simulink model "generator_simulation"  (R2019a)
settings: Solver=FixedStepAuto  StartTime=0.0  StopTime=600  FixedStep=Ts  MaxStep=Ts  RelTol=1e-3
PreLoadFcn:
  | Ts = Ts;
values from neighbouring files (symbols this model uses):
  alpha = 0    [parameters.m]
  Area = 1.13    [parameters.m]
  c_d = 0.5    [parameters.m]
  f = 0.018    [parameters.m]
  g = 9.81    [parameters.m]
  I_initial = v_desired/(R_bx)    (= 0)    [parameters.m]
  Jb = (m_b)*((R_bxb)^2)    (= 41.86125)    [parameters.m]
  Jx = (m_x)*((R_bx)^2)    (= 29.64574716)    [parameters.m]
  m_b = 450    [parameters.m]
  p = 1.204    [parameters.m]
  R_bx = 0.4318    [parameters.m]
  R_bxb = 0.305    [parameters.m]
libraries: powerlib x13, simulink x6
settings Model: EnablePacing=on  Creator=Phuc  LastModifiedBy=Dinh Ngoc Quy
settings SolverCC: AlgebraicLoopSolver=LineSearch
settings DataIOCC: ReturnWorkspaceOutputs=off
settings DebuggingCC: AlgebraicLoopMsg=none  ArithmeticOperatorsInVariantConditions=warning
settings SFSimCC: SimUseLocalCustomCode=off
settings RTWCC: RTWUseLocalCustomCode=off

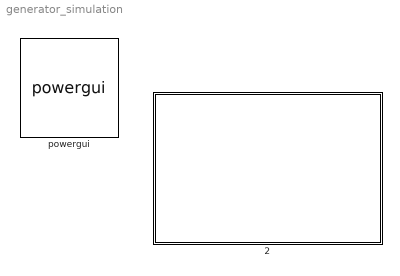
== system generator_simulation ==
  2 : Subsystem
      mask Display:
      | image('motorelec.jpg')
      | port_label('input',1,'w (rad/s)')
  powergui : powerlib/powergui  SimulationMode=Discrete  SampleTime=Ts  frequency=60  Iterations=50  frequencyindice=50  Pbase=100e6  ErrMax=1e-4  UnitsV=kV  UnitsW=MW  buscounter=0  FunctionMessages=off  echomessages=off  EnableUseOfTLC=off  CurrentSourceSwitches=off  DisableSnubberDevices=off  DisableRonSwitches=off  DisableVfSwitches=off  DisplayEquations=off  AutomaticDiscreteSolvers=off  SolverType=Tustin/Backward Euler (TBE)  Interpol=off  ExternalGateDelay=off  methode=off  Ts=100  x0status=blocks  SPID=off  SwTol=0  HookPort=off  NonlinearTolerance=0  nMaxIteration=15  ContinueOnMaxIteration=off  RestoreLinks=warning  ResistiveCurrentMeasurement=off  Frange=[0:2:500]  Ylog=off  Xlog=on  ShowGrid=off  save=off  variable=ZData  structure=0  ZoomFFT=on  StartTime=0.0  cycles=1  DisplayStyle=1  fundamental=60  FreqAxis=off  MaxFrequency=1000  frequencyindicesteady=1  RmsSteady=1  display=off
      settings: SourceProductName=Simscape Electrical

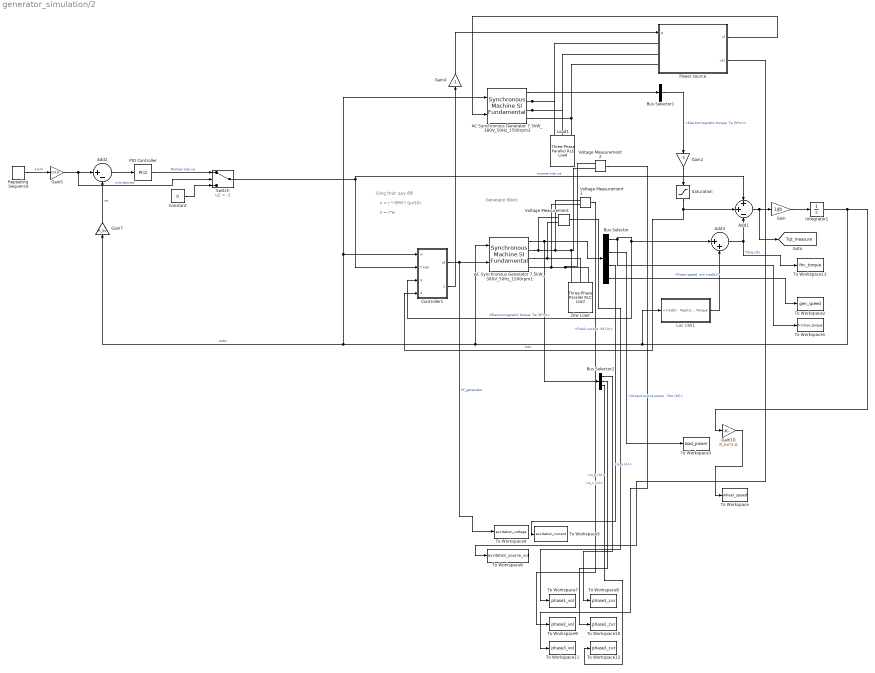
== system generator_simulation/2 ==
  note: Generator Block
  note: Công thức quy đổi
  note: v = r * RPM * (pi/30)
  note: v = r*w
  2kw Load : powerlib/Elements/Three-Phase Parallel RLC Load  LConnTagsString=A|B|C  Configuration=Y (grounded)  NominalVoltage=72  Vabc=[1e3 1e3 1e3]  Vabcp=[1e3 1e3 1e3]  NominalFrequency=50  UnbalancedPower=off  ActivePower=1000  InductivePower=0  CapacitivePower=0  Pabc=[10e3 9e3 11e3]  QLabc=[100 90 110]  QCabc=[100 90 110]  Pabcp=[10e3 9e3 11e3]  QLabcp=[100 90 110]  QCabcp=[100 90 110]  Measurements=None  LoadType=constant Z
      settings: SourceProductName=Simscape Electrical
  AC Synchronous Generator 7.5kW_380V_50Hz_1500rpm1 : powerlib/Machines/Synchronous Machine SI Fundamental  PresetModel=No  MechanicalLoad=Speed w  ShowDetailedParameters=on  RotorType=Salient-pole  Units=SI fundamental parameters  MeasurementBus=off  NominalParameters=[7500 220 50 2]  Stator=[1.62 0.004527 0.1086 0.05175]  Field=[1.208 0.01132]  Dampers2=[ 0.0664, 1.387e-3, 0.0292, 6.896e-4, 7.907e-3, 2.477e-3]  Dampers1=[3.142 0.007334 4.772 0.01015]  Mechanical=[0.0923 0.009 2]  PolePairs=2  InitialConditions="[ 0  0  0  0  0  0  0  0 0]"  SetSaturation=off  Saturation=[695.64,774.7,917.5,1001.6,1082.2,1175.9,1293.6,1430.2,1583.7;9660,10623,12243,13063,13757,14437,15180,15890,16567]  DisplayVfd=off  LoadFlowParameters=[1,0,0,0,0]  TsPowergui=0  TsBlock=-1  IterativeModel=Trapezoidal non iterative  IterativeDiscreteModel=Trapezoidal non iterative  BusType=swing  Pref=0  Qref=0  Qmin=-inf  Qmax=inf  PLF=0  QLF=0
      settings: SourceProductName=Simscape Electrical  SourceProductBaseCode=PS
  AC Synchronous Generator 7.5kW_380V_50Hz_1500rpm2 : powerlib/Machines/Synchronous Machine SI Fundamental  PresetModel=No  MechanicalLoad=Speed w  ShowDetailedParameters=on  RotorType=Salient-pole  Units=SI fundamental parameters  MeasurementBus=off  NominalParameters=[7500 220 50 2]  Stator=[1.62 0.004527 0.1086 0.05175]  Field=[1.208 0.01132]  Dampers2=[ 0.0664, 1.387e-3, 0.0292, 6.896e-4, 7.907e-3, 2.477e-3]  Dampers1=[3.142 0.007334 4.772 0.01015]  Mechanical=[0.0923 0.009 2]  PolePairs=2  InitialConditions="[ 0  0  0  0  0  0  0  0 0]"  SetSaturation=off  Saturation=[695.64,774.7,917.5,1001.6,1082.2,1175.9,1293.6,1430.2,1583.7;9660,10623,12243,13063,13757,14437,15180,15890,16567]  DisplayVfd=off  LoadFlowParameters=[1,0,0,0,0]  TsPowergui=0  TsBlock=-1  IterativeModel=Trapezoidal non iterative  IterativeDiscreteModel=Trapezoidal non iterative  BusType=swing  Pref=0  Qref=0  Qmin=-inf  Qmax=inf  PLF=0  QLF=0
      settings: SourceProductName=Simscape Electrical  SourceProductBaseCode=PS
  Add1 : Sum  Inputs=++-
  Add2 : Sum  Inputs=|+-
  Add3 : Sum  Inputs=|++
  Bus Selector : BusSelector  OutputSignals="Mechanical.Electromagnetic torque  Te (N*m),Output active power   Peo (W),dq0 components.Field current  ifd (A),Mechanical.Rotor speed  wm (rad/s)"
  Bus Selector1 : BusSelector  OutputSignals="Mechanical.Electromagnetic torque  Te (N*m)"
  Bus Selector2 : BusSelector  OutputSignals=Stator current.is_a (A),Stator current.is_b (A),Stator current.is_c (A)
  Constant : Constant  Value=0
  Controller1 : Subsystem
  Gain : Gain  Gain=1/Jb
  Gain10 : Gain  Gain=R_bx*3.6
  Gain2 : Gain  Gain=-1
  Gain4 : Gain  Gain=-1
  Gain5 : Gain  Gain=1/3.6
  Gain7 : Gain  Gain=R_bx
  Integrator1 : Integrator  InitialCondition=I_initial  LimitOutput=on  LowerSaturationLimit=0  ContinuousStateAttributes='velocity'
  Load1 : powerlib/Elements/Three-Phase Parallel RLC Load  LConnTagsString=A|B|C  Configuration=Y (grounded)  NominalVoltage=72  Vabc=[1e3 1e3 1e3]  Vabcp=[1e3 1e3 1e3]  NominalFrequency=50  UnbalancedPower=off  ActivePower=50  InductivePower=0  CapacitivePower=0  Pabc=[10e3 9e3 11e3]  QLabc=[100 90 110]  QCabc=[100 90 110]  Pabcp=[10e3 9e3 11e3]  QLabcp=[100 90 110]  QCabcp=[100 90 110]  Measurements=None  LoadType=constant Z
      settings: SourceProductName=Simscape Electrical
  Luc can1 : Subsystem
  PID Controller : simulink/Continuous/PID Controller  Controller=PI  Form=Ideal  TimeDomain=Discrete-time  SampleTime=-1  IntegratorMethod=Forward Euler  FilterMethod=Forward Euler  ControllerParametersSource=internal  P=435.0333770128  I=0.175017866772017  D=0  UseFilter=on  N=100  TunerSelectOption=Transfer Function Based (PID Tuner App)  InitialConditionSource=internal  InitialConditionForIntegrator=0  InitialConditionForFilter=0  DifferentiatorICPrevScaledInput=0  ExternalReset=none  TrackingMode=off  Kt=1  LimitOutput=off  UpperSaturationLimit=inf  LowerSaturationLimit=-inf  LinearizeAsGain=on  AntiWindupMode=none  Kb=1  POutMin=[]  POutMax=[]  IOutMin=[]  IOutMax=[]  DOutMin=[]  DOutMax=[]  NOutMin=[]  NOutMax=[]  SumOutMin=[]  SumOutMax=[]  SaturationOutMin=[]  SaturationOutMax=[]  PParamMin=[]  PParamMax=[]  IParamMin=[]  IParamMax=[]  DParamMin=[]  DParamMax=[]  NParamMin=[]  NParamMax=[]  KbParamMin=[]  KbParamMax=[]  KtParamMin=[]  KtParamMax=[]  KbOutMin=[]  KbOutMax=[]  KtOutMin=[]  KtOutMax=[]  IntegratorOutMin=[]  IntegratorOutMax=[]  FilterOutMin=[]  FilterOutMax=[]  SumI1OutMin=[]  SumI1OutMax=[]  SumI2OutMin=[]  SumI2OutMax=[]  SumI3OutMin=[]  SumI3OutMax=[]  SumI4OutMin=[]  SumI4OutMax=[]  SumDOutMin=[]  SumDOutMax=[]  DifferentiatorOutMin=[]  DifferentiatorOutMax=[]  FilterDiffOutCoefMin=[]  FilterDiffOutCoefMax=[]  ReciprocalOutMin=[]  ReciprocalOutMax=[]  SumDenOutMin=[]  SumDenOutMax=[]  SumNumOutMin=[]  SumNumOutMax=[]  DivideOutMin=[]  DivideOutMax=[]  IntegratorContinuousStateAttributes=''  IntegratorStateMustResolveToSignalObject=off  IntegratorRTWStateStorageClass=Auto  FilterContinuousStateAttributes=''  FilterStateMustResolveToSignalObject=off  FilterRTWStateStorageClass=Auto  ParallelPVariant=Passthrough  IdealPVariant=InternalParameters  IVariant=InternalParameters  DVariant=Disabled  IntegratorVariant=Discrete  SatVariant=Disabled  AWVariant=Passthrough  PCopyVariant=Disabled  TRVariant=Disabled  FdbkBlocksVariant=Forward  IdealPFdbkVariant=Disabled  SatFdbkVariant=Disabled  DerivativeFilterVariant=Disabled  NVariant=Disabled  NCopyVariant=Disabled_SignalSpec  FilterICVariant=Disabled  IntegratorICVariant=InternalICs  ExternalResetVariant=Disabled  TRSumVariant=Passthrough  SumFdbkVariant=Disabled  SumVariant=Sum_PI
  Power source : Subsystem
  Repeating Sequence : simulink/Sources/Repeating Sequence  rep_seq_t=DriveCycle_time  rep_seq_y=DriveCycle_speed
  Saturation : Saturate  UpperLimit=inf  LowerLimit=0
  Switch : Switch  Criteria=u2 > Threshold  Threshold=-1
  To Workspace : ToWorkspace  VariableName=wheel_speed  SaveFormat=Timeseries  SampleTime=1
  To Workspace1 : ToWorkspace  VariableName=friction_torque  SaveFormat=Timeseries  SampleTime=1
  To Workspace10 : ToWorkspace  VariableName=phase2_cur  SaveFormat=Timeseries  SampleTime=1
  To Workspace11 : ToWorkspace  VariableName=phase3_vol  SaveFormat=Timeseries  SampleTime=1
  To Workspace12 : ToWorkspace  VariableName=phase3_cur  SaveFormat=Timeseries  SampleTime=1
  To Workspace13 : ToWorkspace  VariableName=fric_torque  SaveFormat=Timeseries  SampleTime=1
  To Workspace2 : ToWorkspace  VariableName=gen_speed  SaveFormat=Timeseries  SampleTime=1
  To Workspace3 : ToWorkspace  VariableName=load_power  SaveFormat=Timeseries  SampleTime=1
  To Workspace4 : ToWorkspace  VariableName=excitation_voltage  SaveFormat=Timeseries  SampleTime=1
  To Workspace5 : ToWorkspace  VariableName=excitation_current  SaveFormat=Timeseries  SampleTime=1
  To Workspace6 : ToWorkspace  VariableName=excitation_source_vol  SaveFormat=Timeseries  SampleTime=1
  To Workspace7 : ToWorkspace  VariableName=phase1_vol  SaveFormat=Timeseries  SampleTime=1
  To Workspace8 : ToWorkspace  VariableName=phase1_cur  SaveFormat=Timeseries  SampleTime=1
  To Workspace9 : ToWorkspace  VariableName=phase2_vol  SaveFormat=Timeseries  SampleTime=1
  Voltage Measurement : powerlib/Measurements/Voltage Measurement  PhasorSimulation=off  OutputType=Complex  PSBequivalent=0
      settings: SourceProductName=Simscape Electrical
  Voltage Measurement1 : powerlib/Measurements/Voltage Measurement  PhasorSimulation=off  OutputType=Complex  PSBequivalent=0
      settings: SourceProductName=Simscape Electrical
  Voltage Measurement2 : powerlib/Measurements/Voltage Measurement  PhasorSimulation=off  OutputType=Complex  PSBequivalent=0
      settings: SourceProductName=Simscape Electrical
  tag scope: Tqt_measure=global
  wires:
  Saturation/1 -> Add1/2, Controller1/4(T_motor)  "kéo"
  Integrator1/1 -> Gain10/1, Luc can1/1(v (rad/s)), AC Synchronous Generator 7.5kW_380V_50Hz_1500rpm1/1, Gain7/1, AC Synchronous Generator 7.5kW_380V_50Hz_1500rpm2/1, Controller1/1(w)  "rad/s"
  Gain2/1 -> Saturation/1
  Bus Selector1/1 -> Gain2/1  "<Electromagnetic torque  Te (N*m)>"
  AC Synchronous Generator 7.5kW_380V_50Hz_1500rpm2/1 -> Bus Selector1/1
  Add3/1 -> Add1/3, To Workspace13/1  "Tổng cản"
  Luc can1/1(Resitive Torque) -> Add3/2
  Add1/1 -> [Tqt_measure], Gain/1
  Bus Selector/1 -> Controller1/3(T_measured), Add3/1, To Workspace1/1  "<Electromagnetic torque  Te (N*m)>"
  Gain/1 -> Integrator1/1
  AC Synchronous Generator 7.5kW_380V_50Hz_1500rpm1/1 -> Bus Selector2/1, Bus Selector/1
  Controller1/1(Vf) -> To Workspace4/1, AC Synchronous Generator 7.5kW_380V_50Hz_1500rpm1/2  "Vf_generator"
  Power source/1(vf) -> AC Synchronous Generator 7.5kW_380V_50Hz_1500rpm2/2
  Repeating Sequence/1 -> Gain5/1  "km/h"
  Add2/1 -> PID Controller/1
  Gain7/1 -> Add2/2  "xe"
  Gain5/1 -> Switch/2, Add2/1  "m/s desired"
  Switch/1 -> Add1/1, Controller1/2(T kéo)  "momen kéo xe"
  Constant/1 -> Switch/3
  PID Controller/1 -> Switch/1  "Momen kéo xe"
  Controller1/2(Vf_motor) -> Gain4/1
  Gain4/1 -> Power source/1(g)
  Bus Selector/2 -> To Workspace3/1  "<Output active power   Peo (W)>"
  Gain10/1 -> To Workspace/1
  Bus Selector/3 -> To Workspace5/1  "<Field current  ifd (A)>"
  Power source/2(vf1) -> To Workspace6/1
  Bus Selector2/1 -> To Workspace8/1  "<is_a (A)>"
  Bus Selector2/2 -> To Workspace10/1  "<is_b (A)>"
  Bus Selector2/3 -> To Workspace12/1  "<is_c (A)>"
  Voltage Measurement/1 -> To Workspace7/1
  Voltage Measurement1/1 -> To Workspace9/1
  Voltage Measurement2/1 -> To Workspace11/1
  Bus Selector/4 -> To Workspace2/1  "<Rotor speed  wm (rad/s)>"
  connections:
  AC Synchronous Generator 7.5kW_380V_50Hz_1500rpm2/RConn3 -- Power source/LConn3 -- Load1/LConn3
  AC Synchronous Generator 7.5kW_380V_50Hz_1500rpm2/RConn2 -- Power source/LConn2 -- Load1/LConn2
  AC Synchronous Generator 7.5kW_380V_50Hz_1500rpm2/RConn1 -- Power source/LConn1 -- Load1/LConn1
  AC Synchronous Generator 7.5kW_380V_50Hz_1500rpm1/RConn2 -- Voltage Measurement/LConn2 -- 2kw Load/LConn2
  2kw Load/LConn3 -- Voltage Measurement2/LConn1 -- Voltage Measurement1/LConn2 -- AC Synchronous Generator 7.5kW_380V_50Hz_1500rpm1/RConn3
  AC Synchronous Generator 7.5kW_380V_50Hz_1500rpm1/RConn1 -- Voltage Measurement/LConn1 -- Voltage Measurement1/LConn1 -- Voltage Measurement2/LConn2 -- 2kw Load/LConn1

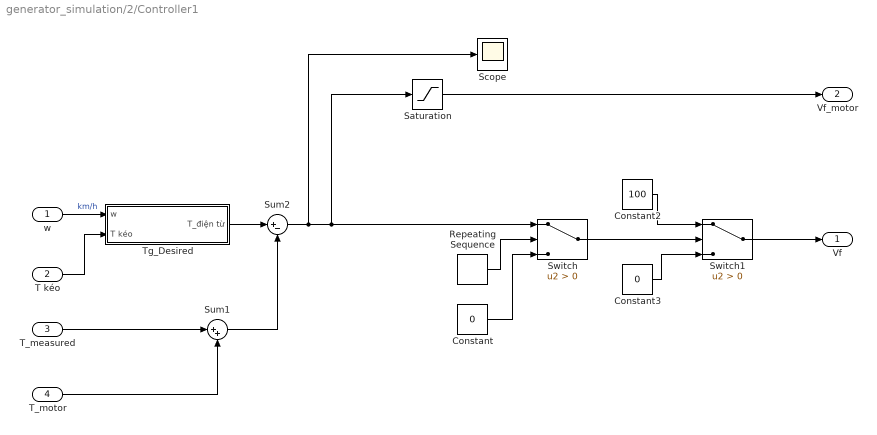
== system generator_simulation/2/Controller1 ==
  w : Inport
  T kéo : Inport  Port=2
  T_measured : Inport  Port=3
  T_motor : Inport  Port=4
  Constant : Constant  Value=0
  Constant2 : Constant  Value=100
  Constant3 : Constant  Value=0
  Repeating Sequence : simulink/Sources/Repeating Sequence  rep_seq_t=DriveCycle_time  rep_seq_y=DriveCycle_speed
  Saturation : Saturate  UpperLimit=0  LowerLimit=-inf
  Scope : Scope
  Sum1 : Sum  Inputs=|++
  Sum2 : Sum  Inputs=|+-
  Switch : Switch  Criteria=u2 > Threshold
  Switch1 : Switch  Criteria=u2 > Threshold
  Tg_Desired : Subsystem
  Vf : Outport
  Vf_motor : Outport  Port=2
  wires:
  Sum1/1 -> Sum2/2
  T_motor/1 -> Sum1/2
  T_measured/1 -> Sum1/1
  Sum2/1 -> Scope/1, Saturation/1, Switch/1
  Tg_Desired/1(T_điện từ) -> Sum2/1
  Switch1/1 -> Vf/1
  Constant3/1 -> Switch1/3
  Constant2/1 -> Switch1/1
  T kéo/1 -> Tg_Desired/2(T kéo)
  w/1 -> Tg_Desired/1(w)  "km/h"
  Constant/1 -> Switch/3
  Switch/1 -> Switch1/2
  Repeating Sequence/1 -> Switch/2
  Saturation/1 -> Vf_motor/1

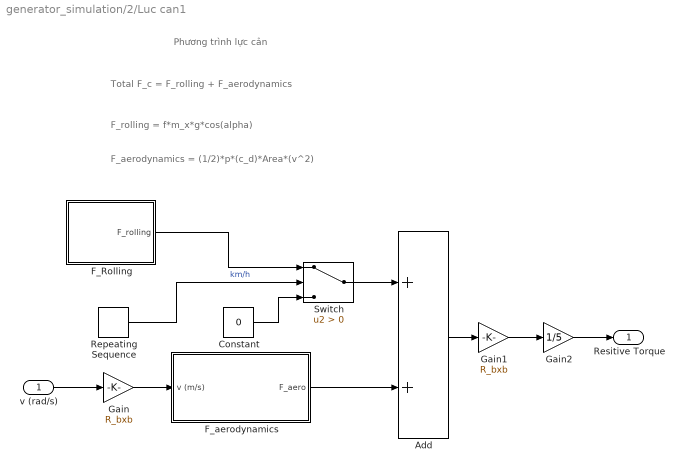
== system generator_simulation/2/Luc can1 ==
  note: Phương trình lực cản
  note: F_aerodynamics = (1/2)*p*(c_d)*Area*(v^2)
  note: F_rolling = f*m_x*g*cos(alpha)
  note: Total F_c = F_rolling + F_aerodynamics
  v (rad/s) : Inport
  Add : Sum
  Constant : Constant  Value=0
  F_Rolling : Subsystem
  F_aerodynamics : Subsystem
  Gain : Gain  Gain=R_bxb
  Gain1 : Gain  Gain=R_bxb
  Gain2 : Gain  Gain=1/5
  Repeating Sequence : simulink/Sources/Repeating Sequence  rep_seq_t=DriveCycle_time  rep_seq_y=DriveCycle_speed
  Switch : Switch  Criteria=u2 > Threshold
  Resitive Torque : Outport
  wires:
  Gain1/1 -> Gain2/1
  Gain/1 -> F_aerodynamics/1(v (m/s))
  Add/1 -> Gain1/1
  v (rad/s)/1 -> Gain/1
  Gain2/1 -> Resitive Torque/1
  F_aerodynamics/1(F_aero) -> Add/2
  Repeating Sequence/1 -> Switch/2  "km/h"
  Constant/1 -> Switch/3
  F_Rolling/1(F_rolling) -> Switch/1
  Switch/1 -> Add/1

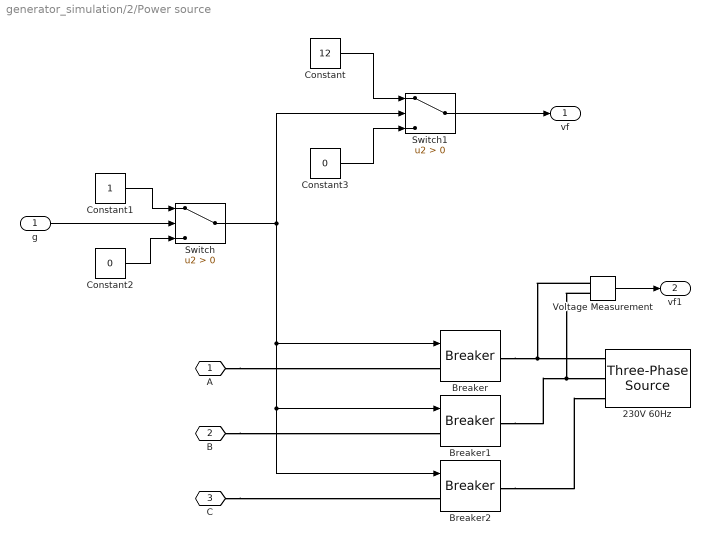
== system generator_simulation/2/Power source ==
  g : Inport
  230V 60Hz : powerlib/Electrical Sources/Three-Phase Source  InternalConnection=Yg  VoltagePhases=off  Voltage=72  PhaseAngle=0  Voltage_phases=[25e3 25e3 25e3]/sqrt(3)  PhaseAngles_phases=[0 -120 +120]  Frequency=50  NonIdealSource=on  SpecifyImpedance=off  Resistance=0.0002  Inductance=0.05e-3  ShortCircuitLevel=100e6  BaseVoltage=72  XRratio=7  BusType=swing  Pref=0  Qref=0  Prefabc=[10e3, 10e3, 10e3]  Qrefabc=[0, 0, 0]  Qmin=-inf  Qmax=inf
      settings: SourceProductName=Simscape Electrical
  Breaker : powerlib/Elements/Breaker  InitialState=0  SwitchingTimes="[1/60  5/60]"  External=on  BreakerResistance=0.01  SnubberResistance=1e6  SnubberCapacitance=inf  Measurements=None  MoreParameters=on  NoBreakLoop=off
      settings: SourceProductName=Simscape Electrical
  Breaker1 : powerlib/Elements/Breaker  InitialState=0  SwitchingTimes="[1/60  5/60]"  External=on  BreakerResistance=0.01  SnubberResistance=1e6  SnubberCapacitance=inf  Measurements=None  MoreParameters=on  NoBreakLoop=off
      settings: SourceProductName=Simscape Electrical
  Breaker2 : powerlib/Elements/Breaker  InitialState=0  SwitchingTimes="[1/60  5/60]"  External=on  BreakerResistance=0.01  SnubberResistance=1e6  SnubberCapacitance=inf  Measurements=None  MoreParameters=on  NoBreakLoop=off
      settings: SourceProductName=Simscape Electrical
  Constant : Constant  Value=12
  Constant1 : Constant
  Constant2 : Constant  Value=0
  Constant3 : Constant  Value=0
  Switch : Switch  Criteria=u2 > Threshold
  Switch1 : Switch  Criteria=u2 > Threshold
  Voltage Measurement : powerlib/Measurements/Voltage Measurement  PhasorSimulation=off  OutputType=Complex  PSBequivalent=0
      settings: SourceProductName=Simscape Electrical
  A : PMIOPort  Side=Left
  B : PMIOPort  Port=2  Side=Left
  C : PMIOPort  Port=3  Side=Left
  vf : Outport
  vf1 : Outport  Port=2
  wires:
  Switch1/1 -> vf/1
  Constant3/1 -> Switch1/3
  Constant/1 -> Switch1/1
  g/1 -> Switch/2
  Constant2/1 -> Switch/3
  Constant1/1 -> Switch/1
  Switch/1 -> Switch1/2, Breaker/1, Breaker1/1, Breaker2/1
  Voltage Measurement/1 -> vf1/1
  connections:
  B/RConn1 -- Breaker1/LConn1
  C/RConn1 -- Breaker2/LConn1
  A/RConn1 -- Breaker/LConn1
  Breaker1/RConn1 -- Voltage Measurement/LConn2 -- 230V 60Hz/RConn2
  Breaker/RConn1 -- Voltage Measurement/LConn1 -- 230V 60Hz/RConn1
  Breaker2/RConn1 -- 230V 60Hz/RConn3

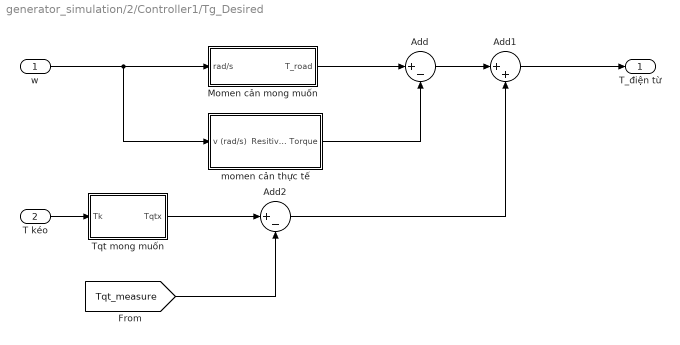
== system generator_simulation/2/Controller1/Tg_Desired ==
  w : Inport
  T kéo : Inport  Port=2
  Add : Sum  Inputs=|+-
  Add1 : Sum  Inputs=|++
  Add2 : Sum  Inputs=|+-
  Momen cản mong muốn : Subsystem
  Tqt mong muốn : Subsystem
  momen cản thực tế : Subsystem
  T_điện từ : Outport
  wires:
  momen cản thực tế/1(Resitive Torque) -> Add/2
  Add1/1 -> T_điện từ/1
  Momen cản mong muốn/1(T_road) -> Add/1
  w/1 -> momen cản thực tế/1(v (rad/s)), Momen cản mong muốn/1(rad/s)
  T kéo/1 -> Tqt mong muốn/1(Tk)
  Tqt mong muốn/1(Tqtx) -> Add2/1
  [Tqt_measure] -> Add2/2
  Add2/1 -> Add1/2
  Add/1 -> Add1/1

== system generator_simulation/2/Luc can1/F_Rolling ==
  Constant : Constant  Value=f
  Constant1 : Constant  Value=m_b
  Constant2 : Constant  Value=g
  Constant3 : Constant  Value=alpha
  Cos : Trigonometry  Operator=cos
  Product1 : Product  Inputs=4
  F_rolling : Outport
  wires:
  Constant2/1 -> Product1/3
  Constant3/1 -> Cos/1
  Product1/1 -> F_rolling/1
  Constant1/1 -> Product1/2
  Cos/1 -> Product1/4
  Constant/1 -> Product1/1

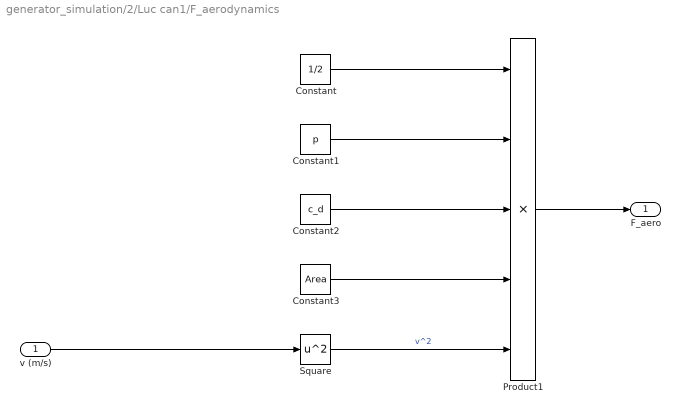
== system generator_simulation/2/Luc can1/F_aerodynamics ==
  v (m/s) : Inport
  Constant : Constant  Value=1/2
  Constant1 : Constant  Value=p
  Constant2 : Constant  Value=c_d
  Constant3 : Constant  Value=Area
  Product1 : Product  Inputs=5
  Square : Math  Operator=square  RndMeth=Zero  SaturateOnIntegerOverflow=on
  F_aero : Outport
  wires:
  v (m/s)/1 -> Square/1
  Constant/1 -> Product1/1
  Constant3/1 -> Product1/4
  Constant1/1 -> Product1/2
  Constant2/1 -> Product1/3
  Square/1 -> Product1/5  "v^2"
  Product1/1 -> F_aero/1

== system generator_simulation/2/Controller1/Tg_Desired/Momen cản mong muốn ==
  rad/s : Inport
  Luc can : Subsystem
  R_bánh xe bệ2 : Gain  Gain=R_bx
  R_bánh xe bệ3 : Gain  Gain=R_bx
  T_road : Outport
  wires:
  Luc can/1(Resitive Force) -> R_bánh xe bệ3/1
  R_bánh xe bệ3/1 -> T_road/1
  R_bánh xe bệ2/1 -> Luc can/1(v)  "v (m/s)"
  rad/s/1 -> R_bánh xe bệ2/1

== system generator_simulation/2/Controller1/Tg_Desired/Tqt mong muốn ==
  Tk : Inport
  Gain1 : Gain  Gain=1/Jx
  Integrator1 : Integrator  InitialCondition=I_initial  LimitOutput=on  LowerSaturationLimit=0  ContinuousStateAttributes='velocity'
  Sum1 : Sum  Inputs=|+-
  momen cản : Subsystem
  Tqtx : Outport
  wires:
  momen cản/1(Resitive Torque) -> Sum1/2  "Tc"
  Integrator1/1 -> momen cản/1(v (rad/s))  "v(rad/s)"
  Sum1/1 -> Tqtx/1, Gain1/1  "ma"
  Tk/1 -> Sum1/1
  Gain1/1 -> Integrator1/1  "dv/dt"

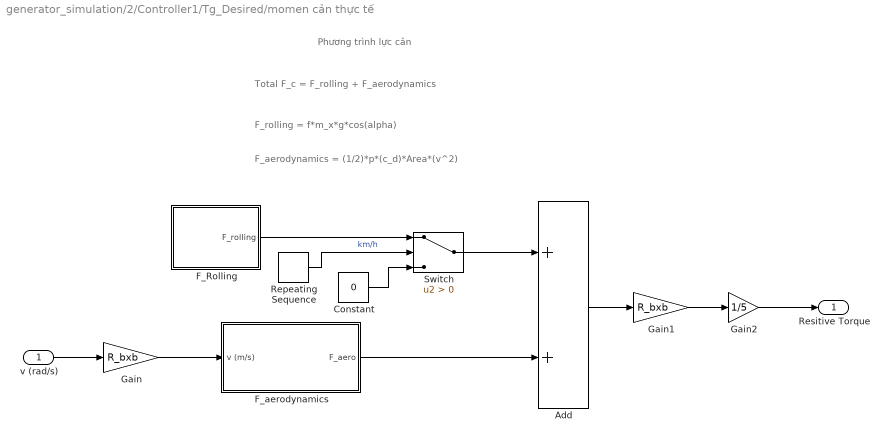
== system generator_simulation/2/Controller1/Tg_Desired/momen cản thực tế ==
  note: Phương trình lực cản
  note: F_aerodynamics = (1/2)*p*(c_d)*Area*(v^2)
  note: F_rolling = f*m_x*g*cos(alpha)
  note: Total F_c = F_rolling + F_aerodynamics
  v (rad/s) : Inport
  Add : Sum
  Constant : Constant  Value=0
  F_Rolling : Subsystem
  F_aerodynamics : Subsystem
  Gain : Gain  Gain=R_bxb
  Gain1 : Gain  Gain=R_bxb
  Gain2 : Gain  Gain=1/5
  Repeating Sequence : simulink/Sources/Repeating Sequence  rep_seq_t=DriveCycle_time  rep_seq_y=DriveCycle_speed
  Switch : Switch  Criteria=u2 > Threshold
  Resitive Torque : Outport
  wires:
  Gain1/1 -> Gain2/1
  Gain/1 -> F_aerodynamics/1(v (m/s))
  Add/1 -> Gain1/1
  v (rad/s)/1 -> Gain/1
  F_aerodynamics/1(F_aero) -> Add/2
  Gain2/1 -> Resitive Torque/1
  F_Rolling/1(F_rolling) -> Switch/1
  Repeating Sequence/1 -> Switch/2  "km/h"
  Constant/1 -> Switch/3
  Switch/1 -> Add/1

== system generator_simulation/2/Controller1/Tg_Desired/Momen cản mong muốn/Luc can ==
  note: Total F_c = F_rolling + F_aerodynamics
  note: F_rolling = f*m_x*g*cos(alpha)
  note: F_aerodynamics = (1/2)*p*(c_d)*Area*(v^2)
  note: Phương trình lực cản
  v : Inport
  Add : Sum
  F_Rolling : Subsystem
  F_aerodynamics : Subsystem
  Resitive Force : Outport
  wires:
  F_aerodynamics/1(F_aero) -> Add/2
  Add/1 -> Resitive Force/1
  v/1 -> F_aerodynamics/1(v (m/s))
  F_Rolling/1(F_rolling) -> Add/1

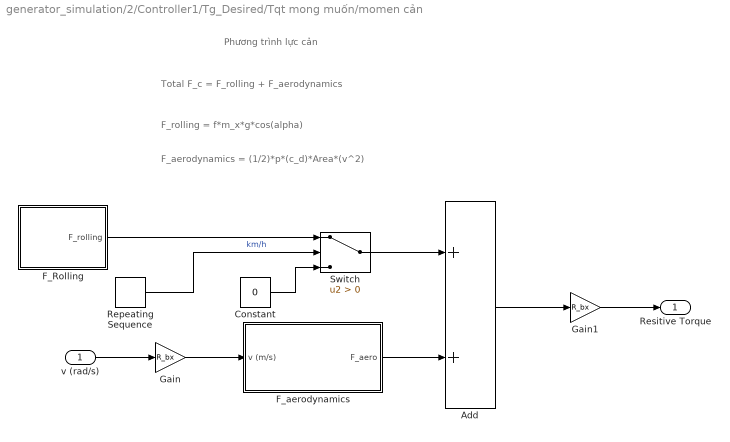
== system generator_simulation/2/Controller1/Tg_Desired/Tqt mong muốn/momen cản ==
  note: Total F_c = F_rolling + F_aerodynamics
  note: F_rolling = f*m_x*g*cos(alpha)
  note: F_aerodynamics = (1/2)*p*(c_d)*Area*(v^2)
  note: Phương trình lực cản
  v (rad/s) : Inport
  Add : Sum
  Constant : Constant  Value=0
  F_Rolling : Subsystem
  F_aerodynamics : Subsystem
  Gain : Gain  Gain=R_bx
  Gain1 : Gain  Gain=R_bx
  Repeating Sequence : simulink/Sources/Repeating Sequence  rep_seq_t=DriveCycle_time  rep_seq_y=DriveCycle_speed
  Switch : Switch  Criteria=u2 > Threshold
  Resitive Torque : Outport
  wires:
  F_aerodynamics/1(F_aero) -> Add/2
  v (rad/s)/1 -> Gain/1
  Add/1 -> Gain1/1
  Gain1/1 -> Resitive Torque/1
  Gain/1 -> F_aerodynamics/1(v (m/s))
  Repeating Sequence/1 -> Switch/2  "km/h"
  Constant/1 -> Switch/3
  F_Rolling/1(F_rolling) -> Switch/1
  Switch/1 -> Add/1

== system generator_simulation/2/Controller1/Tg_Desired/momen cản thực tế/F_Rolling ==
  Constant : Constant  Value=f
  Constant1 : Constant  Value=m_b
  Constant2 : Constant  Value=g
  Constant3 : Constant  Value=alpha
  Cos : Trigonometry  Operator=cos
  Product1 : Product  Inputs=4
  F_rolling : Outport
  wires:
  Constant2/1 -> Product1/3
  Constant3/1 -> Cos/1
  Product1/1 -> F_rolling/1
  Constant1/1 -> Product1/2
  Cos/1 -> Product1/4
  Constant/1 -> Product1/1

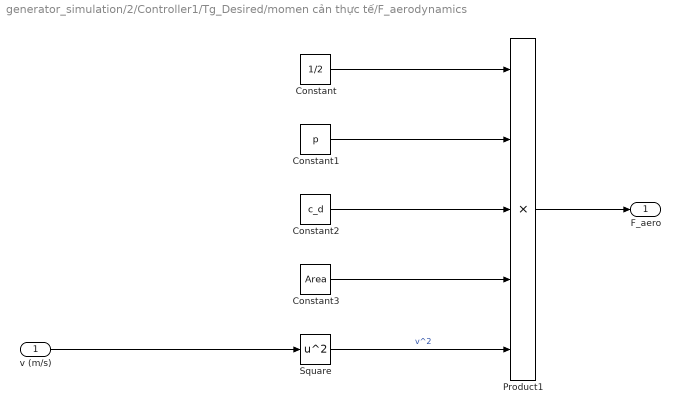
== system generator_simulation/2/Controller1/Tg_Desired/momen cản thực tế/F_aerodynamics ==
  v (m/s) : Inport
  Constant : Constant  Value=1/2
  Constant1 : Constant  Value=p
  Constant2 : Constant  Value=c_d
  Constant3 : Constant  Value=Area
  Product1 : Product  Inputs=5
  Square : Math  Operator=square  RndMeth=Zero  SaturateOnIntegerOverflow=on
  F_aero : Outport
  wires:
  v (m/s)/1 -> Square/1
  Constant/1 -> Product1/1
  Constant3/1 -> Product1/4
  Constant1/1 -> Product1/2
  Constant2/1 -> Product1/3
  Square/1 -> Product1/5  "v^2"
  Product1/1 -> F_aero/1

== system generator_simulation/2/Controller1/Tg_Desired/Momen cản mong muốn/Luc can/F_Rolling ==
  Constant : Constant  Value=f
  Constant1 : Constant  Value=m_b
  Constant2 : Constant  Value=g
  Constant3 : Constant  Value=alpha
  Cos : Trigonometry  Operator=cos
  Product1 : Product  Inputs=4
  F_rolling : Outport
  wires:
  Constant2/1 -> Product1/3
  Constant3/1 -> Cos/1
  Product1/1 -> F_rolling/1
  Constant1/1 -> Product1/2
  Cos/1 -> Product1/4
  Constant/1 -> Product1/1

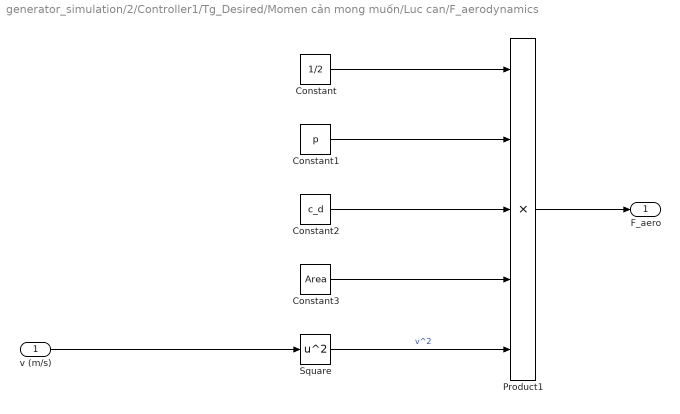
== system generator_simulation/2/Controller1/Tg_Desired/Momen cản mong muốn/Luc can/F_aerodynamics ==
  v (m/s) : Inport
  Constant : Constant  Value=1/2
  Constant1 : Constant  Value=p
  Constant2 : Constant  Value=c_d
  Constant3 : Constant  Value=Area
  Product1 : Product  Inputs=5
  Square : Math  Operator=square  RndMeth=Zero  SaturateOnIntegerOverflow=on
  F_aero : Outport
  wires:
  Product1/1 -> F_aero/1
  Square/1 -> Product1/5  "v^2"
  Constant2/1 -> Product1/3
  Constant1/1 -> Product1/2
  Constant3/1 -> Product1/4
  Constant/1 -> Product1/1
  v (m/s)/1 -> Square/1

== system generator_simulation/2/Controller1/Tg_Desired/Tqt mong muốn/momen cản/F_Rolling ==
  Constant : Constant  Value=f
  Constant1 : Constant  Value=m_b
  Constant2 : Constant  Value=g
  Constant3 : Constant  Value=alpha
  Cos : Trigonometry  Operator=cos
  Product1 : Product  Inputs=4
  F_rolling : Outport
  wires:
  Constant2/1 -> Product1/3
  Constant3/1 -> Cos/1
  Product1/1 -> F_rolling/1
  Constant1/1 -> Product1/2
  Cos/1 -> Product1/4
  Constant/1 -> Product1/1

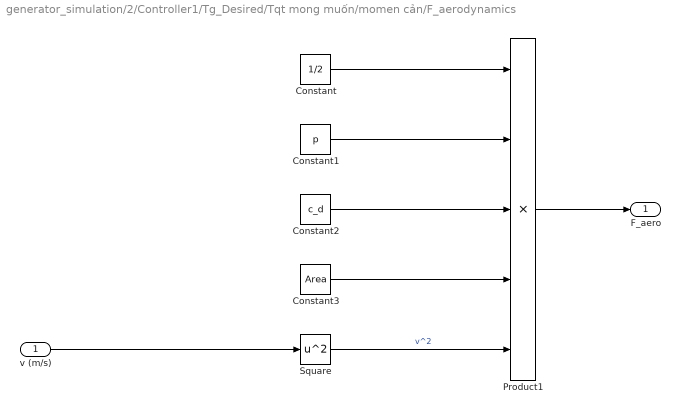
== system generator_simulation/2/Controller1/Tg_Desired/Tqt mong muốn/momen cản/F_aerodynamics ==
  v (m/s) : Inport
  Constant : Constant  Value=1/2
  Constant1 : Constant  Value=p
  Constant2 : Constant  Value=c_d
  Constant3 : Constant  Value=Area
  Product1 : Product  Inputs=5
  Square : Math  Operator=square  RndMeth=Zero  SaturateOnIntegerOverflow=on
  F_aero : Outport
  wires:
  Product1/1 -> F_aero/1
  Square/1 -> Product1/5  "v^2"
  Constant2/1 -> Product1/3
  Constant1/1 -> Product1/2
  Constant3/1 -> Product1/4
  Constant/1 -> Product1/1
  v (m/s)/1 -> Square/1
